simulink model "cranePlantSimulation"  (R2020b)
settings: Solver=ode4  StartTime=0.0  StopTime=50  FixedStep=0.002  RelTol=1e-3  EnableMultiTasking=on
InitFcn:
  | %% Motor
  | % Resistance
  | Rm = 8.4;
  | % Current-torque (N-m/A)
  | kt = 0.042;
  | % Back-emf constant (V-s/rad)
  | km = 0.042;
  | %
  | %% Rotary Arm
  | % Mass (kg)
  | Mr = 0.095;
  | % Total length (m)
  | Lr = 0.085;
  | % Moment of inertia about pivot (kg-m^2)
  | Jr = Mr*Lr^2/12;
  | % Equivalent Viscous Damping Coefficient (N-m-s/rad)
  | Dr = 0.0015;
  | % Dr = 0.001;
  | %
  | %% Pendulum Link
  | % Mass (kg)
  | Mp = 0.024;
  | % Total length (m)
  | Lp = 0.129;
  | % Moment of inertia about pivot (kg-m^2)
  | Jp = Mp*Lp^2/12;
  | % Equivalent Viscous Damping Coefficient (N-m-s/rad)
  | Dp = 0.0005;
  | Dp = 0.0004;
  | % Gravity Constant
  | g = 9.81;
  | %
  | %% Get system equations
  | % Find Total Inertia
  | Jt = Jr*Jp + Mp*(Lp/2)^2*Jr + Jp*Mp*Lr^2;
  | 
  | % % State Space Representation
  | A = [0 0 1 0;
  |      0 0 0 1;
  |      0 Mp^2*(Lp/2)^2*Lr*g/Jt -Dr*(Jp+Mp*(Lp/2)^2)/Jt Mp*(Lp/2)*Lr*Dp/Jt;
  |      0 -Mp*g*(Lp/2)*(Jr+Mp*Lr^2)/Jt Mp*(Lp/2)*Lr*Dr/Jt -Dp*(Jr+Mp*Lr^2)/Jt];
  | %
  | % A = [0          0           1           0;
  | %      0          0           0           1;
  | %      -k/c0,  c2*c4/c3/c0, -Dr/c0,Dp*c2/c3/c0;
  | %      c2*k/c5, -c1*c4/c5, c2*Dr/c5, c1*Dp/c5];
  | 
  | 
  | B = [0; 0; (Jp+Mp*(Lp/2)^2)/Jt; -Mp*(Lp/2)*Lr/Jt];
  | %
  | % B = [0;
  | %      0;
  | %      c3*kt/Rm;
  | %      -c2*kt/Rm/c5];
  | 
  | C = eye(2,4);
  | D = zeros(2,1);
  | 
  | % Add actuator dynamics
  | B = km * B / Rm;
  | A(3,3) = A(3,3) - km*km/Rm*B(3);
  | A(4,3) = A(4,3) - km*km/Rm*B(4);
  | 
  | sys = ss(A,B,C,D);
  | 
  | 
  | 
  | 
  | c1 = (Mp*Lr^2 + Jr); % theta acceleration coefficient (i.e. inertia term) in dynamics
  | c2 = 0.5*Mp*Lr*Lp; % alpha acceleration coefficient in dynamics
  | c3 = Jp + 0.25*Mp*Lp^2;
  | c4 = 0.5*Mp*Lp*9.81;
  | 
  | c5 = c2*(c2 + c1*c3/c2);
  | c0 = c1 + c2^2/c3;
  | 
  | omega = 10; % a filter parameter
  | den = [1 Dr/c1 omega]; % denominator of filter
  | 
  | %% model spring term in theta
  | 
  | % modify equations to deal with spring constant in theta due to encoder cable
  | k = 0.0008; % [Nm/rad] what i think it is
  | % k = 130;
  | A(3,1) = -c3*k/Jt; % I THINK C3 IS THE CORRECT MULTIPLIER.
  | A(4,1) = c2*k/Jt;
  | 
  | 
  | [r,p] = residue([-Dr/c1 -omega],den); % partial fraction expansion for alpha terms, used to generate first order filters
  | % [r,p] = residue([1 0 0],den); % partial fraction expansion for alpha terms, used to generate first order filters
  | 
  | p0 = 10000; % estimation gain
  | 
  | 
  | %% Kalman filter
  | 
  | % DONT TOUCH?
  | Qn = 0.5^2; % Qn is one row because it's the covariance of the disturbance w, which is scalar
  | Rn = diag([(pi/2048)^2, (pi/2048)^2]);
  | 
  | 
  | kalmansys = ss(A, [B B], C, 0);
  | 
  | [kest, L, P] = kalman(sys,Qn,Rn);
  | % poles = [-33,-33, -49, -49];
  | % L = place(A',C',poles).';
  | 
  | eig(A-L*C);
settings Model: ExtModeTrigDuration=25001  Creator=felix  LastModifiedBy=nick
settings SolverCC: PositivePriorityOrder=on
settings DataIOCC: LimitDataPoints=on  SaveFormat=Array  ReturnWorkspaceOutputs=off
settings OptimizationCC: LifeSpan=inf
settings DebuggingCC: SolverPrmCheckMsg=warning  AllowSymbolicDim=off  SFUnexpectedBacktrackingDiag=warning  SFNoUnconditionalDefaultTransitionDiag=warning  SFExecutionAtInitializationDiag=none  ArithmeticOperatorsInVariantConditions=warning
settings HardwareCC: ProdBitPerPointer=32  ProdBitPerSizeT=32  ProdBitPerPtrDiffT=32  ProdLargestAtomicFloat=None  ProdIntDivRoundTo=Undefined  ProdEndianess=Unspecified  ProdWordSize=32  ProdHWDeviceType=32-bit Generic
settings ModelReferenceCC: PropagateSignalLabelsOutOfModel=off
settings SFSimCC: SimUseLocalCustomCode=off  CustomCodeUndefinedFunction=UseInterfaceOnly
settings RTWCC: Description=QUARC Win64 Target  SystemTargetFile=quarc_win64.tlc  TemplateMakefile=quarc_default_tmf  RTWUseLocalCustomCode=off
settings CodeAppCC: StateflowObjectComments=on
settings STFCustomTargetCC: TargetPreCompLibLocation=C:\PROGRA~3\QUARC\lib\2015b\win64\release  CombineOutputUpdateFcns=on  CPPClassGenCompliant=off  GRTInterface=off
settings GRTTargetCC: TargetPreCompLibLocation=C:\PROGRA~3\QUARC\lib\2015b\win64\release  TargetLangStandard=C89/C90 (ANSI)  ParMdlRefBuildCompliant=off  CompOptLevelCompliant=off  MatFileLogging=off  CPPClassGenCompliant=off  UseToolchainInfoCompliant=off  ExtMode=on  ExtModeMexFile=quarc_comm
settings ConfigComp: CovMetricSettings=dw  CovSaveCumulativeToWorkspaceVar=on  CovSaveSingleToWorkspaceVar=on  CovExternalEMLEnable=off  CovSFcnEnable=off
settings SimscapeCC: SimscapeNormalizeSystem=off

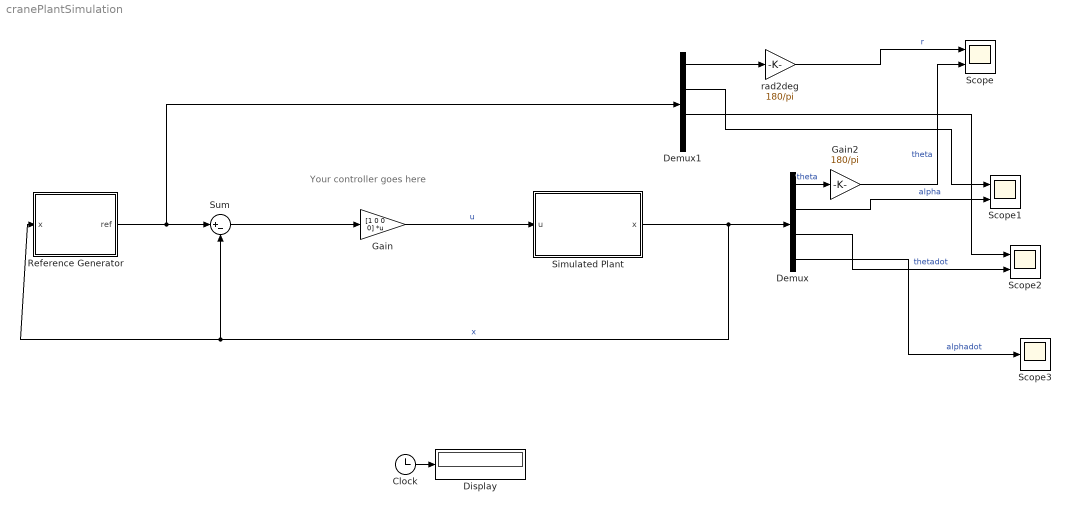
== system cranePlantSimulation ==
  note: Your controller goes here
  Clock : Clock
  Demux : Demux
  Demux1 : Demux
  Display : Display
  Gain : Gain  Gain=[1 0 0 0]  Multiplication=Matrix(K*u)
  Gain2 : Gain  Gain=180/pi
  Reference Generator : Subsystem
  Scope : Scope  NumInputPorts=2
  Scope1 : Scope  NumInputPorts=2
  Scope2 : Scope  NumInputPorts=2
  Scope3 : Scope
  Simulated Plant : Subsystem
  Sum : Sum  Inputs=|+-
  rad2deg : Gain  Gain=180/pi
  wires:
  Simulated Plant/1(x) -> Reference Generator/1(x), Sum/2, Demux/1  "x"
  Gain/1 -> Simulated Plant/1(u)  "u"
  Sum/1 -> Gain/1
  Demux/1 -> Gain2/1  "theta"
  Demux/2 -> Scope1/2  "alpha"
  Demux/3 -> Scope2/2  "thetadot"
  Demux/4 -> Scope3/1  "alphadot"
  Demux1/1 -> rad2deg/1
  Gain2/1 -> Scope/2  "theta"
  rad2deg/1 -> Scope/1  "r"
  Clock/1 -> Display/1
  Reference Generator/1(ref) -> Sum/1, Demux1/1
  Demux1/2 -> Scope1/1
  Demux1/3 -> Scope2/1

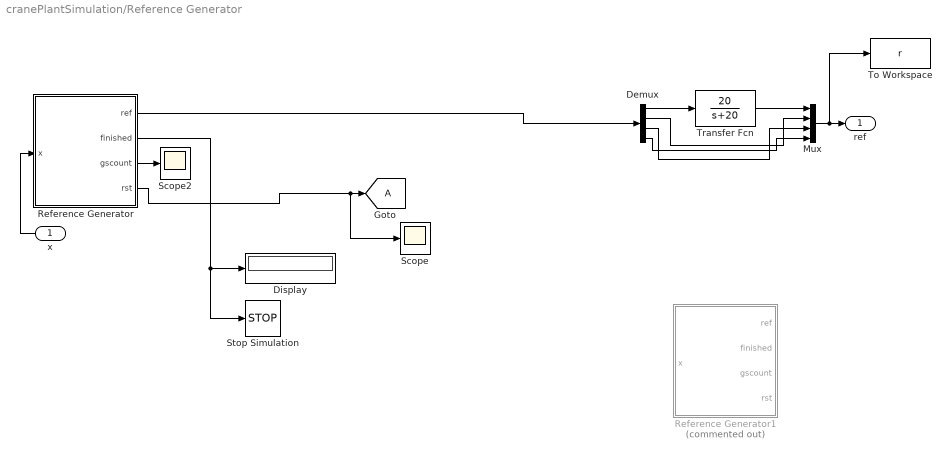
== system cranePlantSimulation/Reference Generator ==
  x : Inport
  Demux : Demux
  Display : Display
  Mux : Mux
  Reference Generator : MATLAB Function  TreatAsAtomicUnit=on  SystemSampleTime=0.002
  Reference Generator1 : MATLAB Function  Commented=on  TreatAsAtomicUnit=on  SystemSampleTime=0.002
  Scope : Scope
  Scope2 : Scope
  Stop Simulation : Stop
  To Workspace : ToWorkspace  VariableName=r  SaveFormat=Structure With Time  SampleTime=0.002
  Transfer Fcn : TransferFcn  Numerator=20  Denominator=[1 20]
  ref : Outport
  tag scope: A=global
  wires:
  Reference Generator/2(finished) -> Stop Simulation/1, Display/1
  Reference Generator/1(ref) -> Demux/1
  Reference Generator/3(gscount) -> Scope2/1
  x/1 -> Reference Generator/1(x)
  Reference Generator/4(rst) -> Scope/1, [A]
  Demux/1 -> Transfer Fcn/1
  Transfer Fcn/1 -> Mux/1
  Demux/2 -> Mux/2
  Demux/3 -> Mux/3
  Demux/4 -> Mux/4
  Mux/1 -> To Workspace/1, ref/1

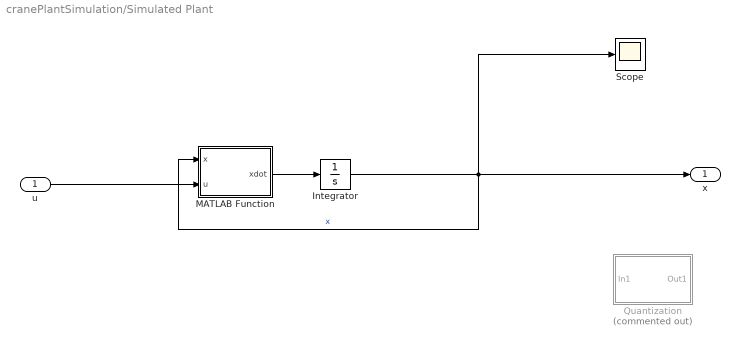
== system cranePlantSimulation/Simulated Plant ==
  u : Inport
  Integrator : Integrator  InitialCondition=[0;0;0;0]
  MATLAB Function : MATLAB Function  TreatAsAtomicUnit=on
  Quantization : Subsystem  Commented=on
  Scope : Scope
  x : Outport
  wires:
  u/1 -> MATLAB Function/2(u)
  Integrator/1 -> x/1, Scope/1, MATLAB Function/1(x)  "x"
  MATLAB Function/1(xdot) -> Integrator/1

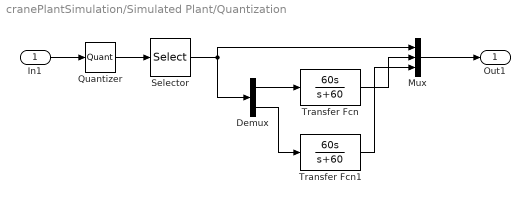
== system cranePlantSimulation/Simulated Plant/Quantization ==
  In1 : Inport
  Demux : Demux  Outputs=2
  Mux : Mux  Inputs=3
  Quantizer : Quantizer  QuantizationInterval=2*pi/2048
  Selector : Selector  InputPortWidth=4  IndexOptions=Index vector (dialog)  Indices=[1 2]  OutputSizes=1
  Transfer Fcn : TransferFcn  Numerator=[60 0]  Denominator=[1 60]
  Transfer Fcn1 : TransferFcn  Numerator=[60 0]  Denominator=[1 60]
  Out1 : Outport
  wires:
  Transfer Fcn1/1 -> Mux/3
  In1/1 -> Quantizer/1
  Demux/1 -> Transfer Fcn/1
  Transfer Fcn/1 -> Mux/2
  Selector/1 -> Mux/1, Demux/1
  Quantizer/1 -> Selector/1
  Demux/2 -> Transfer Fcn1/1
  Mux/1 -> Out1/1

== matlab function cranePlantSimulation/Reference Generator/Reference Generator ==
  data: x input size=4; ref output; finished output; gscount output; rst output
function [ref, finished, gscount,rst] = referenceGenerator(x)
%#codegen
%     coder.allowpcode('REFGEN');
    [ref, finished, gscount, rst] = REFGEN(x);
end

== matlab function cranePlantSimulation/Reference Generator/Reference Generator1 ==
  data: x input size=4; ref output; finished output; gscount output; rst output
function [ref, finished, gscount,rst] = REFGEN(x)
%#codegen
%% Crane Reference Generator: For AMME3500 Lab 3 (2016)
% 
% Generates three `waypoints' for the crane's horizontal linkage. When the
% state is settled close to the reference at close to zero velocity, the
% next waypoint is given (the change is a step change). When all the waypoints 
% have been reached, then the task is finished.
%
% Let q1 be the horizontal linkage, and q2 be the vertical (unactuated)
% linkage on the pendulum.
%
%
% Input: 
% x         [4x1] [q1; q2; q1dot; q2dot] (rad and rad/s)
%
% Output:
% ref       [1x1] q1 reference position (rad)
%

%% Declare variables
% Persistent variables
persistent n 
% persistent holdcheck
persistent goodSteps % counts how many timesteps tolerances have been satisfied for
persistent done

if(isempty(n))
    n = 1; % start at first waypoint
    done = false;
end
if(isempty(goodSteps))
    goodSteps = 1;
end

    ref = zeros(4,1);

    % Local variables
    waypoints = [30; -60; 45; -30]*pi/180; % reference waypoints
    posTolArm = 1*pi/180; % [rad] position tolerance
    posTolPend = posTolArm;
    velTolArm = 0.1; % [rad/s] velocity tolerance
    velTolPend = 0.1; % [rad/s] basically KF tolerance.

    %% Detect successful arrival at waypoint
%     
% %     reset count if tolerances violated
%     if(~done) % only check for arrival if not done
%         if(abs(waypoints(n)-x(1)) <= posTolArm) % q1 arrived
%             if(abs(x(2)) <= posTolPend) % q2 pointing straight down
%                 if(abs(x(3)) <= velTolArm && abs(x(4)) <= velTolPend) % q1 and q2 stationary
%                     count = count + 1; % increment count if everything satisifed this timestep
%                 else
% %                     count = 1;
%                 end
%             else
% %                 count = 1;
%             end
%         else
% %             count = 1;
%         end
%     end

    if (abs(waypoints(n)-x(1)) <= posTolArm) && (abs(x(2)) <= posTolPend) && (abs(x(3)) <= velTolArm) && (abs(x(4)) <= velTolPend) % q1 and q2 stationary
        goodSteps = goodSteps + 1; % increment count if everything satisifed this timestep
    else
        goodSteps = 1; % reset if tolerances breached
    end

    rst = false;
    %% detect successful completion of waypoint
    holdTime = 3; % number of seconds that tolerances have to be satisfied for it to count
    if goodSteps >= holdTime/0.002 
        rst = true;
        n = n + 1;
        if n > length(waypoints);
            done = true;
        end
    end
    
    gscount = goodSteps;
%% Output reference
if(~done)
    ref(1) = waypoints(n);
    finished = done;
else
    ref(1) = waypoints(end);
    finished = done;
end

== matlab function cranePlantSimulation/Simulated Plant/MATLAB Function ==
  data: x input size=4; u input size=1; xdot output size=4
function xdot = fcn(x,u)

    xdot = dyn(x,u);


end
